simulink model "controller_for_carsimDIYROS"  (R2021a)
settings: Solver=VariableStepAuto  StartTime=0.0  StopTime=15  RelTol=1e-2
values from neighbouring files (symbols this model uses):
  Vx = 15    [controller_setup.m]
libraries: robotlib x23, Solver_SF x1, simulink_extras x1, simulink x1
settings Model: Creator=dekunw  LastModifiedBy=chnwa
settings SolverCC: AlgebraicLoopSolver=LineSearch
settings DebuggingCC: SFMachineParentedDataDiag=warning

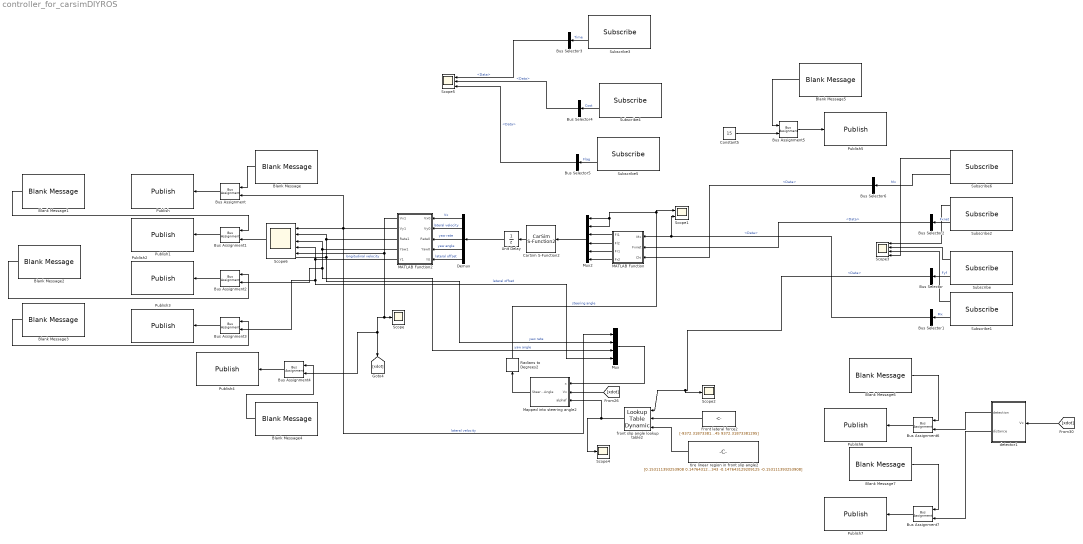
== system controller_for_carsimDIYROS ==
  Blank Message{,1..7} (8 alike) : robotlib/Blank Message  messageClass=Message  entityType=std_msgs/Float64  messageType=std_msgs/Float64  SampleTime=inf  legacyBusStruct=off
  Bus Assignment{,1..7} (8 alike) : BusAssignment  AssignedSignals=Data
  Bus Selector{,1..6} (7 alike) : BusSelector  OutputSignals=Data
  CarSim S-Function2 : Solver_SF/CarSim S-Function2  Priority=1  VehicleCode=i_i  SIMFILE=simfile.sim
      settings: AttributesFormatString=Vehicle Code: %<VehicleCode>
  Constant5 : Constant  Value=15
  Demux : Demux  Outputs=5
  Front lateral force2 : Constant  Value="[-9372.31873381295\t-9371.87234490745\t-9368.75632133124\t-9360.32413915416\t-9343.95286497491\t-9317.04140044534\t-9277.00875557097\t-9221.29234898623\t-9147.34633344744\t-9052.63994482675\t-8934.65587292915\t-8790.88865249026\t-8618.84307274575\t-8416.03260399439\t-8179.97783960505\t-7908.20495194422\t-7598.24416072470\t-7247.62821229778\t-6853.89086843106\t-6414.56540313147\t-5927.18310608872\t-5389.27179132790\t-4798.35430967129\t-4151.94706361935\t-3447.55852326814\t-2682.68774188626\t-1854.82286977838\t-961.439665063923\t0\t961.439665063923\t1854.82286977838\t2682.68774188626\t3447.55852326814\t4151.94706361935\t4798.35430967129\t5389.27179132790\t5927.18310608872\t6414.56540313147\t6853.89086843106\t7247.62821229778\t7598.24416072470\t7908.20495194422\t8179.97783960505\t8416.03260399439\t8618.84307274575\t8790.88865249026\t8934.65587292915\t9052.63994482675\t9147.34633344744\t9221.29234898623\t9277.00875557097\t9317.04140044534\t9343.95286497491\t9360.32413915416\t9368.75632133124\t9371.87234490745\t9372.31873381295]"
  MATLAB Function : MATLAB Function  TreatAsAtomicUnit=on
  MATLAB Function2 : MATLAB Function  TreatAsAtomicUnit=on
  Mapped into steering angle2 : MATLAB Function  TreatAsAtomicUnit=on
  Mux : Mux
  Mux2 : Mux  Inputs=6
  Publish : robotlib/Publish  topicSource=Specify your own  topic=/states1  messageType=std_msgs/Float64  legacyBusStruct=off  messageQueueLength=1
  Publish1 : robotlib/Publish  topicSource=Specify your own  topic=/states2  messageType=std_msgs/Float64  legacyBusStruct=off  messageQueueLength=1
  Publish2 : robotlib/Publish  topicSource=Specify your own  topic=/states3  messageType=std_msgs/Float64  legacyBusStruct=off  messageQueueLength=1
  Publish3 : robotlib/Publish  topicSource=Specify your own  topic=/states4  messageType=std_msgs/Float64  legacyBusStruct=off  messageQueueLength=1
  Publish4 : robotlib/Publish  topicSource=Specify your own  topic=/Vx  messageType=std_msgs/Float64  legacyBusStruct=off  messageQueueLength=1
  Publish5 : robotlib/Publish  topicSource=Specify your own  topic=/Vset  messageType=std_msgs/Float64  legacyBusStruct=off  messageQueueLength=1
  Publish6 : robotlib/Publish  topicSource=Specify your own  topic=/Detection  messageType=std_msgs/Float64  legacyBusStruct=off  messageQueueLength=1
  Publish7 : robotlib/Publish  topicSource=Specify your own  topic=/Distance  messageType=std_msgs/Float64  legacyBusStruct=off  messageQueueLength=1
  Radians to Degrees2 : simulink_extras/Transformations/Radians to Degrees
  Scope : Scope
  Scope1 : Scope  NumInputPorts=2
  Scope2 : Scope
  Scope3 : Scope  NumInputPorts=4
  Scope4 : Scope
  Scope5 : Scope  NumInputPorts=3
  Scope6 : Scope  NumInputPorts=5
  Subscribe : robotlib/Subscribe  topicSource=Specify your own  topic=/ControlInput1  messageType=std_msgs/Float64  SampleTime=-1  legacyBusStruct=off  messageQueueLength=1
  Subscribe1 : robotlib/Subscribe  topicSource=Specify your own  topic=/ControlInput2  messageType=std_msgs/Float64  SampleTime=-1  legacyBusStruct=off  messageQueueLength=1
  Subscribe2 : robotlib/Subscribe  topicSource=Specify your own  topic=/Fxnet  messageType=std_msgs/Float64  SampleTime=-1  legacyBusStruct=off  messageQueueLength=1
  Subscribe3 : robotlib/Subscribe  topicSource=Specify your own  topic=/Time  messageType=std_msgs/Float64  SampleTime=-1  legacyBusStruct=off  messageQueueLength=1
  Subscribe4 : robotlib/Subscribe  topicSource=Specify your own  topic=/CostValue  messageType=std_msgs/Float64  SampleTime=-1  legacyBusStruct=off  messageQueueLength=1
  Subscribe5 : robotlib/Subscribe  topicSource=Specify your own  topic=/Flag  messageType=std_msgs/Float64  SampleTime=-1  legacyBusStruct=off  messageQueueLength=1
  Subscribe6 : robotlib/Subscribe  topicSource=Specify your own  topic=/ControlInput2  messageType=std_msgs/Float64  SampleTime=-1  legacyBusStruct=off  messageQueueLength=1
  Unit Delay : UnitDelay  InitialCondition=[54 0 0 0 0]'  SampleTime=-1  HasFrameUpgradeWarning=on
  detector1 : Subsystem
  front slip angle lookup table2 : simulink/Lookup Tables/Lookup Table Dynamic  LookUpMeth=Interpolation-Use End Values  OutDataType=fixdt('double')  OutScaling=[]  OutputDataTypeScalingMode=Specify via dialog  OutDataTypeStr=double  DoSatur=off
  tire linear region in front slip angle2 : Constant  Value="[0.153111393253908\t0.147643129209125\t0.142174865164343\t0.136706601119560\t0.131238337074778\t0.125770073029996\t0.120301808985213\t0.114833544940431\t0.109365280895648\t0.103897016850866\t0.0984287528060835\t0.0929604887613011\t0.0874922247165187\t0.0820239606717363\t0.0765556966269539\t0.0710874325821714\t0.0656191685373890\t0.0601509044926066\t0.0546826404478242\t0.0492143764030418\t0.0437461123582594\t0.0382778483134769\t0.0328095842686945\t0.0273413202239121\t0.0218730561791297\t0.0164047921343473\t0.0109365280895648\t0.00546826404478242\t0\t-0.00546826404478242\t-0.0109365280895648\t-0.0164047921343473\t-0.0218730561791297\t-0.0273413202239121\t-0.0328095842686945\t-0.0382778483134769\t-0.0437461123582594\t-0.0492143764030418\t-0.0546826404478242\t-0.0601509044926066\t-0.0656191685373890\t-0.0710874325821714\t-0.0765556966269539\t-0.0820239606717363\t-0.0874922247165187\t-0.0929604887613011\t-0.0984287528060835\t-0.103897016850866\t-0.109365280895648\t-0.114833544940431\t-0.120301808985213\t-0.125770073029996\t-0.131238337074778\t-0.136706601119560\t-0.142174865164343\t-0.147643129209125\t-0.153111393253908]"
  wires:
  Bus Selector1/1 -> MATLAB Function/1(Mx), Scope1/2  "<Data>"
  tire linear region in front slip angle2/1 -> front slip angle lookup table2/3
  [xdot] -> Mapped into steering angle2/2(Vx)
  Bus Selector/1 -> Scope2/1, front slip angle lookup table2/1  "<Data>"
  Front lateral force2/1 -> front slip angle lookup table2/2
  Radians to Degrees2/1 -> Mux2/2, Mux2/1, Scope1/1  "steering angle"
  front slip angle lookup table2/1 -> Scope4/1, Mapped into steering angle2/3(alphaf)
  Mapped into steering angle2/1(SteeringAngle) -> Radians to Degrees2/1
  MATLAB Function2/2(Vy1) -> Bus Assignment/2, Scope6/1, Mux/1  "lateral velocity"
  MATLAB Function2/3(Rate1) -> Scope6/2, Mux/2, Bus Assignment1/2  "yaw rate"
  MATLAB Function2/5(Y1) -> Mux/4, Bus Assignment3/2, Scope6/4  "lateral offset"
  Mux2/1 -> CarSim S-Function2/1
  CarSim S-Function2/1 -> Unit Delay/1
  MATLAB Function2/1(Vx1) -> [xdot], Bus Assignment4/2, Scope/1, Scope6/5  "longitudinal velocity"
  MATLAB Function2/4(Yaw1) -> Scope6/3, Mux/3, Bus Assignment2/2  "yaw angle"
  MATLAB Function/1(Fl1) -> Mux2/3
  MATLAB Function/2(Fl2) -> Mux2/4
  MATLAB Function/3(Fr1) -> Mux2/5
  MATLAB Function/4(Fr2) -> Mux2/6
  Constant5/1 -> Bus Assignment5/2
  Bus Assignment5/1 -> Publish5/1
  Blank Message5/1 -> Bus Assignment5/1
  Blank Message1/1 -> Bus Assignment1/1
  Blank Message4/1 -> Bus Assignment4/1
  Bus Assignment3/1 -> Publish3/1
  Blank Message2/1 -> Bus Assignment2/1
  Blank Message3/1 -> Bus Assignment3/1
  Blank Message/1 -> Bus Assignment/1
  Bus Assignment1/1 -> Publish1/1
  Bus Assignment4/1 -> Publish4/1
  Bus Assignment2/1 -> Publish2/1
  Bus Assignment/1 -> Publish/1
  Subscribe1/1 -> Scope3/3
  Subscribe2/2 -> Bus Selector2/1  "Fxnet"
  Subscribe/2 -> Bus Selector/1  "Fyf"
  Subscribe2/1 -> Scope3/1
  Subscribe/1 -> Scope3/2
  Subscribe1/2 -> Bus Selector1/1  "Mx"
  Bus Selector2/1 -> MATLAB Function/2(Fxnet)  "<Data>"
  Mux/1 -> Mapped into steering angle2/1(x)
  Bus Assignment6/1 -> Publish6/1
  Blank Message6/1 -> Bus Assignment6/1
  detector1/1(detection) -> Bus Assignment6/2
  Bus Assignment7/1 -> Publish7/1
  Blank Message7/1 -> Bus Assignment7/1
  detector1/2(distance) -> Bus Assignment7/2
  Subscribe3/2 -> Bus Selector3/1  "Time"
  Subscribe4/2 -> Bus Selector4/1  "Cost"
  Subscribe5/2 -> Bus Selector5/1  "Flag"
  Bus Selector3/1 -> Scope5/1  "<Data>"
  Bus Selector4/1 -> Scope5/2  "<Data>"
  Bus Selector5/1 -> Scope5/3  "<Data>"
  Unit Delay/1 -> Demux/1
  Demux/1 -> MATLAB Function2/1(Vx0)  "Vx"
  Demux/2 -> MATLAB Function2/2(Vy0)  "lateral velocity"
  Demux/3 -> MATLAB Function2/3(Rate0)  "yaw rate"
  Demux/4 -> MATLAB Function2/4(Yaw0)  "yaw angle"
  Demux/5 -> MATLAB Function2/5(Y0)  "lateral offset"
  [xdot] -> detector1/1(Vx)
  Subscribe6/2 -> Bus Selector6/1  "Mx"
  Subscribe6/1 -> Scope3/4
  Bus Selector6/1 -> MATLAB Function/3(Chi)  "<Data>"

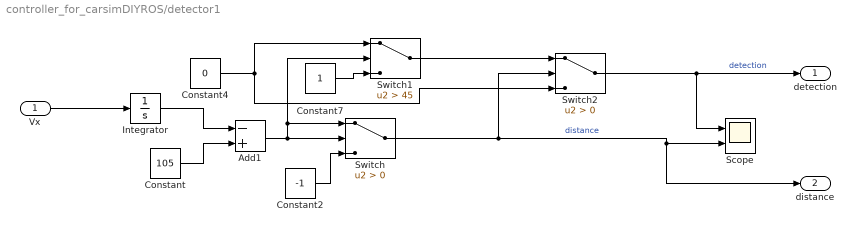
== system controller_for_carsimDIYROS/detector1 ==
  Vx : Inport
  Add1 : Sum  Inputs=-+
  Constant : Constant  Value=105
  Constant2 : Constant  Value=-1
  Constant4 : Constant  Value=0
  Constant7 : Constant
  Integrator : Integrator
  Scope : Scope  NumInputPorts=2
  Switch : Switch  Criteria=u2 > Threshold
  Switch1 : Switch  Criteria=u2 > Threshold  Threshold=45
  Switch2 : Switch  Criteria=u2 > Threshold
  detection : Outport
  distance : Outport  Port=2
  wires:
  Constant2/1 -> Switch/3
  Constant4/1 -> Switch2/3, Switch1/1
  Vx/1 -> Integrator/1
  Integrator/1 -> Add1/1
  Switch/1 -> Switch2/2, Scope/2, distance/1  "distance"
  Constant7/1 -> Switch1/3
  Add1/1 -> Switch1/2, Switch/1, Switch/2
  Switch1/1 -> Switch2/1
  Constant/1 -> Add1/2
  Switch2/1 -> Scope/1, detection/1  "detection"

== matlab function controller_for_carsimDIYROS/MATLAB Function2 ==
  data: Vx0 input; Vx1 output; Vy0 input; Rate0 input; Yaw0 input; Y0 input; Vy1 output; Rate1 output; Yaw1 output; Y1 output
function [Vx1,Vy1,Rate1,Yaw1,Y1] = fcn(Vx0,Vy0,Rate0,Yaw0,Y0)
Vx1=0.277778*Vx0;
Vy1=0.277778*Vy0;
Rate1=Rate0/180*pi;
Yaw1=Yaw0/180*pi;
Y1=Y0;

== matlab function controller_for_carsimDIYROS/Mapped into steering angle2 ==
  data: x input; Vx input; alphaf input; SteeringAngle output
function SteeringAngle = fcn(x,Vx, alphaf)

lf = 1.11;  % distance from front axle to the mass center

Vy = x(1); %lateral velocity
r = x(2);  %yaw rate
SteeringAngle = Vy/Vx+lf*r/Vx-alphaf;

== matlab function controller_for_carsimDIYROS/MATLAB Function ==
  data: Fl1 output; Mx input; Fl2 output; Fxnet input; Fr1 output; Fr2 output; Chi input
function [Fl1,Fl2,Fr1,Fr2] = fcn(Mx,Fxnet,Chi)
Eta_e=0.5; % the ratio of the allocated brakes on the front axle when Chi=1
Eta_f=0.7; % the ratio of the allocated brakes on the front axle when Chi=0
Eta=Eta_f-Chi*(Eta_f-Eta_e);
w = 1.875; % the width of the car

Fwf = zeros(2,1);
Fwr = zeros(2,1);

if Mx > 0
    Fwf(1) = Fxnet/2+0;
    Fwf(2) = Fxnet/2-Eta*2*Mx/w;
    Fwr(1) = 0;
    Fwr(2) = -(1-Eta)*2*Mx/w;
elseif Mx < 0
    Fwf(1) = Fxnet/2+Eta*2*Mx/w;
    Fwf(2) = Fxnet/2+0;
    Fwr(1) = (1-Eta)*2*Mx/w;
    Fwr(2) = 0;
else
    Fwf(1) = Fxnet/2+0;
    Fwf(2) = Fxnet/2+0;
    Fwr(1) = 0;
    Fwr(2) = 0;
end
Fl1 = Fwf(1);
Fl2 = Fwr(1);
Fr1 = Fwf(2);
Fr2 = Fwr(2);
